simulink model "v2_2_S1"  (R2017a)
settings: Solver=VariableStepAuto  StartTime=0.0  StopTime=20  RelTol=1e-3
values from neighbouring files (symbols this model uses):
  TracebackDepth = 64    [v2_2_Hm.m]    (also in v2_2_S3m.m; v2_2_Sm.m)
libraries: commdigbbndpm3 x3, commcnvcod2 x2, commblkintrlv2 x2, commchan3 x1, commrandsrc3 x1, commsink2 x1, dspquant2 x1
settings Model: Creator=DELL  LastModifiedBy=DELL

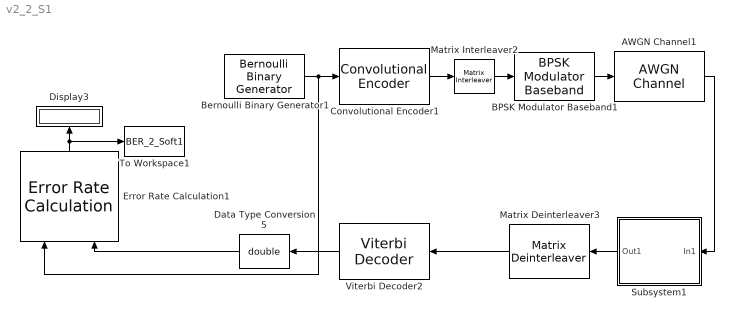
== system v2_2_S1 ==
  AWGN Channel1 : commchan3/AWGN Channel  InputProcessing=Columns as channels (frame based)  seed=113  noiseMode="Signal to noise ratio  (Eb/No)"  EbNodB=EbN0  EsNodB=1  SNRdB=10  bitsPerSym=1  Ps=1  Tsym=1e-5  variance=1
  BPSK Modulator Baseband1 : commdigbbndpm3/BPSK Modulator Baseband  Ph=0  outDtype=double  outWordLen=16  outUDDataType=sfix(16)  outFracLenMode=Best precision  outFracLen=15  outDataTypeStr=double  outLastDataTypeStr=double
  Bernoulli Binary Generator1 : commrandsrc3/Bernoulli Binary Generator  ProbabilityOfZero=0.5  SeedSource=Auto  Seed=0  SampleTime=1e-5  SamplesPerFrame=SamplesPerFrame  OutputDataType=double  SimulateUsing=Interpreted execution
  Convolutional Encoder1 : commcnvcod2/Convolutional Encoder  trellis=poly2trellis(9, [561 753])  opMode=Continuous  DelayedResetAction=off  hasIniStPort=off  hasFinStPort=off  usePuncVector=off  punctureVector=[1; 1; 0; 1; 0; 1]  reset=Unused parameter value
      settings: SourceProductName=Communications System Toolbox  SourceProductBaseCode=CM
  Data Type Conversion5 : DataTypeConversion  OutDataTypeStr=double
  Display3 : Display
  Error Rate Calculation1 : commsink2/Error Rate Calculation  N=TracebackDepth  st_delay=0  cp_mode=Entire frame  subframe=[]  PMode=Port  WsName=ErrorVec  RsMode2=off  stop=off  numErr=100  maxBits=1e6
  Matrix Deinterleaver3 : commblkintrlv2/Matrix Deinterleaver  Nrows=Rows  Ncols=Cols
      settings: SourceProductName=Communications System Toolbox  SourceProductBaseCode=CM
  Matrix Interleaver2 : commblkintrlv2/Matrix Interleaver  Nrows=Rows  Ncols=Cols
      settings: SourceProductName=Communications System Toolbox  SourceProductBaseCode=CM
  Subsystem1 : Subsystem
      mask Display: disp('Soft-Output\nBPSK\nDemodulator')
  To Workspace1 : ToWorkspace  VariableName=BER_2_Soft1  SampleTime=-1
      settings: MaxDataPoints=1
  Viterbi Decoder2 : commcnvcod2/Viterbi Decoder  trellis=poly2trellis(9, [561 753])  isPunctured=off  punctureVector=[1; 1; 0; 1; 0; 1]  erasures=off  dectype=Soft decision  nsdecb=8  runSigValErrCheck=off  tbdepth=TracebackDepth  opmode=Continuous  reset=off  delayedResetAction=off  smWordLength=16  outDataType=Inherit via internal rule
      settings: SourceProductName=Communications System Toolbox  SourceProductBaseCode=CM
  wires:
  Bernoulli Binary Generator1/1 -> Error Rate Calculation1/1, Convolutional Encoder1/1
  Convolutional Encoder1/1 -> Matrix Interleaver2/1
  BPSK Modulator Baseband1/1 -> AWGN Channel1/1
  Viterbi Decoder2/1 -> Data Type Conversion5/1
  Subsystem1/1(Out1) -> Matrix Deinterleaver3/1
  Matrix Deinterleaver3/1 -> Viterbi Decoder2/1
  AWGN Channel1/1 -> Subsystem1/1(In1)
  Data Type Conversion5/1 -> Error Rate Calculation1/2
  Error Rate Calculation1/1 -> To Workspace1/1, Display3/1
  Matrix Interleaver2/1 -> BPSK Modulator Baseband1/1

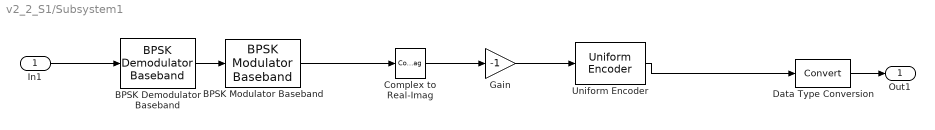
== system v2_2_S1/Subsystem1 ==
  In1 : Inport
  BPSK Demodulator Baseband : commdigbbndpm3/BPSK Demodulator Baseband  DecType=Hard decision  VarSource=Dialog  Variance=1  Ph=0  outDtype=Inherit via internal rule  derotateFactorWordLen=16  derotateFactorDataTypeStr=Inherit: Same word length as input  derotateFactorLastDataTypeStr=Inherit: Same word length as input
  BPSK Modulator Baseband : commdigbbndpm3/BPSK Modulator Baseband  Ph=0  outDtype=double  outWordLen=16  outUDDataType=sfix(16)  outFracLenMode=Best precision  outFracLen=15  outDataTypeStr=double  outLastDataTypeStr=double
  Complex to Real-Imag : ComplexToRealImag  Output=Real
  Data Type Conversion : DataTypeConversion  SaturateOnIntegerOverflow=on  RndMeth=Zero
  Gain : Gain  Gain=-1  SaturateOnIntegerOverflow=on  OutDataTypeStr=Inherit: Same as input  ParamDataTypeStr=Inherit: Same as input
  Uniform Encoder : dspquant2/Uniform Encoder  peak=1  bits=8  otype=Unsigned integer
      settings: SourceProductName=DSP System Toolbox
  Out1 : Outport
  wires:
  Uniform Encoder/1 -> Data Type Conversion/1
  Gain/1 -> Uniform Encoder/1
  Data Type Conversion/1 -> Out1/1
  BPSK Modulator Baseband/1 -> Complex to Real-Imag/1
  BPSK Demodulator Baseband/1 -> BPSK Modulator Baseband/1
  In1/1 -> BPSK Demodulator Baseband/1
  Complex to Real-Imag/1 -> Gain/1
